simulink model "DUS"  (R2020a)
settings: Solver=FixedStepDiscrete  StartTime=0.0  StopTime=10.0  FixedStep=0.01  RelTol=1e-3
libraries: simulink x2
settings Model: Creator=xreno  LastModifiedBy=xreno

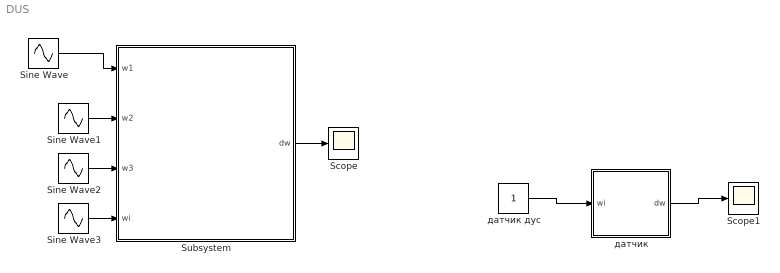
== system DUS ==
  Scope : Scope
  Scope1 : Scope
  Sine Wave{,1..3} (4 alike) : Sin  SampleTime=0
  Subsystem : Subsystem
  датчик : Subsystem
  датчик дус : Constant
  wires:
  Sine Wave/1 -> Subsystem/1(w1)
  Sine Wave3/1 -> Subsystem/4(wi)
  Sine Wave2/1 -> Subsystem/3(w3)
  Sine Wave1/1 -> Subsystem/2(w2)
  Subsystem/1(dw) -> Scope/1
  датчик/1(dw) -> Scope1/1
  датчик дус/1 -> датчик/1(wi)

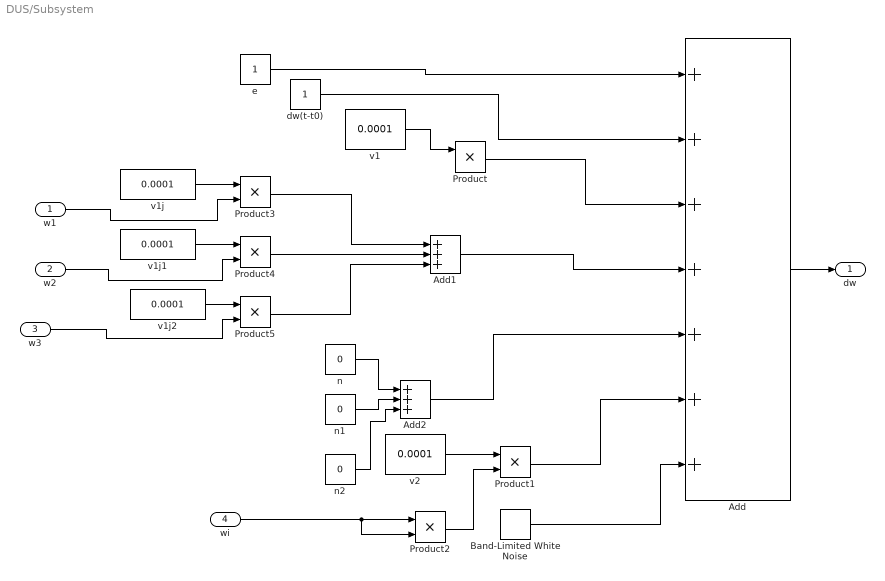
== system DUS/Subsystem ==
  w1 : Inport
  w2 : Inport  Port=2
  w3 : Inport  Port=3
  wi : Inport  Port=4
  Add : Sum  Inputs=+++++++
  Add1 : Sum  Inputs=+++
  Add2 : Sum  Inputs=+++
  Band-Limited White Noise : simulink/Sources/Band-Limited White Noise  Cov=[0.00002]  Ts=0.01  seed=[23341]
  Product{,1..5} (6 alike) : Product
  dw(t-t0) : Constant
  e : Constant
  n : Constant  Value=0
  n1 : Constant  Value=0
  n2 : Constant  Value=0
  v1 : Constant  Value=0.0001
  v1j : Constant  Value=0.0001
  v1j1 : Constant  Value=0.0001
  v1j2 : Constant  Value=0.0001
  v2 : Constant  Value=0.0001
  dw : Outport
  wires:
  e/1 -> Add/1
  dw(t-t0)/1 -> Add/2
  Product1/1 -> Add/6
  Band-Limited White Noise/1 -> Add/7
  v2/1 -> Product1/1
  n/1 -> Add2/1
  Product2/1 -> Product1/2
  v1j2/1 -> Product5/1
  n1/1 -> Add2/2
  Product3/1 -> Add1/1
  Product4/1 -> Add1/2
  Product/1 -> Add/3
  v1/1 -> Product/1
  n2/1 -> Add2/3
  Product5/1 -> Add1/3
  Add2/1 -> Add/5
  v1j1/1 -> Product4/1
  wi/1 -> Product2/2, Product2/1
  Add1/1 -> Add/4
  v1j/1 -> Product3/1
  Add/1 -> dw/1
  w1/1 -> Product3/2
  w2/1 -> Product4/2
  w3/1 -> Product5/2

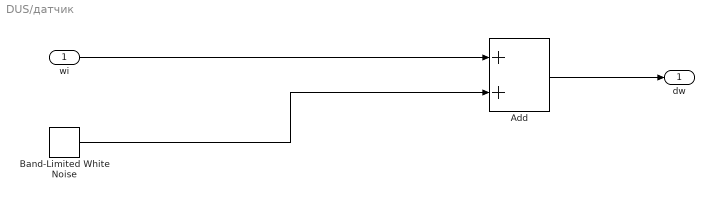
== system DUS/датчик ==
  wi : Inport
  Add : Sum
  Band-Limited White Noise : simulink/Sources/Band-Limited White Noise  Cov=[0.00002]  Ts=0.01  seed=[23341]
  dw : Outport
  wires:
  Band-Limited White Noise/1 -> Add/2
  wi/1 -> Add/1
  Add/1 -> dw/1
